simulink model "capitol3pb1"  (R2013a)
settings: Solver=ode45  StartTime=0.0  StopTime=7200  RelTol=1e-3
undefined symbols (not defined in the file): des, gcbh
settings Model: Creator=user  LastModifiedBy=user

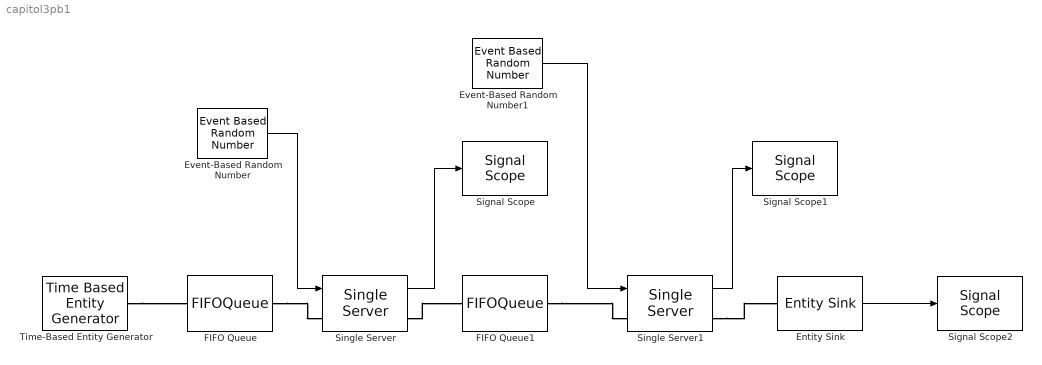
== system capitol3pb1 ==
  Entity Sink : EntitySink  StatNumberArrived=on
  Event-Based Random Number : EventBasedRandomNumber  Distribution=Uniform  minUnif=20  maxUnif=40
  Event-Based Random Number1 : EventBasedRandomNumber  Distribution=Uniform  minUnif=120  maxUnif=240
  FIFO Queue : FIFOQueue
  FIFO Queue1 : FIFOQueue
  Signal Scope : SignalScope  LoadFcn=des.scope.CallbackSupport('seLoadFcn',gcbh)  StartFcn=des.scope.CallbackSupport('seStartFcn',gcbh)  StopFcn=des.scope.CallbackSupport('seStopFcn',gcbh)
      settings: CopyFcn=des.scope.CallbackSupport('seCopyFcn',gcbh)  DeleteFcn=des.scope.CallbackSupport('seDeleteFcn',gcbh)  PreSaveFcn=des.scope.CallbackSupport('sePreSaveFcn',gcbh)  NameChangeFcn=des.scope.CallbackSupport('seNameChangeFcn',gcbh)  OpenFcn=des.scope.CallbackSupport('seOpenFcn',gcbh)
  Signal Scope1 : SignalScope  LoadFcn=des.scope.CallbackSupport('seLoadFcn',gcbh)  StartFcn=des.scope.CallbackSupport('seStartFcn',gcbh)  StopFcn=des.scope.CallbackSupport('seStopFcn',gcbh)
      settings: CopyFcn=des.scope.CallbackSupport('seCopyFcn',gcbh)  DeleteFcn=des.scope.CallbackSupport('seDeleteFcn',gcbh)  PreSaveFcn=des.scope.CallbackSupport('sePreSaveFcn',gcbh)  NameChangeFcn=des.scope.CallbackSupport('seNameChangeFcn',gcbh)  OpenFcn=des.scope.CallbackSupport('seOpenFcn',gcbh)
  Signal Scope2 : SignalScope  LoadFcn=des.scope.CallbackSupport('seLoadFcn',gcbh)  StartFcn=des.scope.CallbackSupport('seStartFcn',gcbh)  StopFcn=des.scope.CallbackSupport('seStopFcn',gcbh)
      settings: CopyFcn=des.scope.CallbackSupport('seCopyFcn',gcbh)  DeleteFcn=des.scope.CallbackSupport('seDeleteFcn',gcbh)  PreSaveFcn=des.scope.CallbackSupport('sePreSaveFcn',gcbh)  NameChangeFcn=des.scope.CallbackSupport('seNameChangeFcn',gcbh)  OpenFcn=des.scope.CallbackSupport('seOpenFcn',gcbh)
  Single Server : SingleServer  ServiceTimeFrom=Signal port t  StatAverageWait=on
      settings: OutputPortMap=o4
  Single Server1 : SingleServer  ServiceTimeFrom=Signal port t  StatAverageWait=on
      settings: OutputPortMap=o4
  Time-Based Entity Generator : TimeBasedEntityGenerator  Distribution=Uniform  Minimum=60  Maximum=180
  wires:
  Event-Based Random Number/1 -> Single Server/1
  Single Server/1 -> Signal Scope/1
  Event-Based Random Number1/1 -> Single Server1/1
  Single Server1/1 -> Signal Scope1/1
  Entity Sink/1 -> Signal Scope2/1
  connections:
  Time-Based Entity Generator/RConn1 -- FIFO Queue/LConn1
  FIFO Queue/RConn1 -- Single Server/LConn1
  Single Server/RConn1 -- FIFO Queue1/LConn1
  FIFO Queue1/RConn1 -- Single Server1/LConn1
  Single Server1/RConn1 -- Entity Sink/LConn1
